simulink model "VTOL_renewal"  (R2023b)
settings: configuration reference "VTOLConfiguration" (kept outside this file)
undefined symbols (not defined in the file): CityMission, control, controlParams, ControlSampleTime, CriticalTiltAngle, DiscIntNeverNeededParam, env, F, FixedWingMission, flightState, FSState, FWControlParams, FWTrimSpeed, HoverMission, iniRoll, initPitch, iniYaw, Light, MIL, R_LOOKAHEAD, ReferenceFilterDen, ReferenceFilterNum, tilt_max, tilt_trim, tiltIni, TiltScheduleRate, TransitionMission, uavParam, vIni, Vt, w_trim, WindDownRate, windVel, xGround, yGround, zGround
libraries: slpidlib x56, simulink x6, uavalgslib x6, mbdriLib x4, aerolibasang x2, aerolibwind2 x2, shared6dof x1, sharedtransform x1, simulink_extras x1, sim3dlib x1, uavsim3dlib x1, uavutilslib x1
(part 2 of 8)

== system VTOL_renewal/Digital Twin/Ground Truth Bus ==
  Ve : Inport
  Xe : Inport  Port=2
  Euler : Inport  Port=3
  DCMbe : Inport  Port=4
  Vb : Inport  Port=5
  pqr : Inport  Port=6
  Abb : Inport  Port=7
  Abe : Inport  Port=8
  RotorParams : Inport  Port=9
  AirData : Inport  Port=10
  Bus Creator : BusCreator  Inputs=13
  Bus Selector : BusSelector  OutputSignals=airspeed
  Direction Cosine Matrix to Quaternions : sharedtransform/Direction Cosine Matrix  to Quaternions  aMode=0  action=None  tolerance=eps(2)
      settings: LibrarySourceBlock=|
      | aerolibtransform2/Direction Cosine Matrix
      | to Quaternions
  MATLAB Function1 : MATLAB Function  TreatAsAtomicUnit=on
  Ground Truth : Outport
  wires:
  pqr/1 -> Bus Creator/6
  Xe/1 -> Bus Creator/2
  Bus Creator/1 -> Ground Truth/1
  DCMbe/1 -> Direction Cosine Matrix to Quaternions/1, Bus Creator/4
  Euler/1 -> Bus Creator/3
  Vb/1 -> Bus Creator/5
  Abb/1 -> Bus Creator/7
  AirData/1 -> Bus Selector/1
  Bus Selector/1 -> Bus Creator/9  "<airspeed>"
  Direction Cosine Matrix to Quaternions/1 -> Bus Creator/10  "q"
  RotorParams/1 -> Bus Creator/8  "RotorParameters"
  Abe/1 -> Bus Creator/11  "Abe"
  MATLAB Function1/2(gndSpeed) -> Bus Creator/13  "gndspeed"
  MATLAB Function1/1(course) -> Bus Creator/12  "course"
  Ve/1 -> MATLAB Function1/1(vxyz), Bus Creator/1

== system VTOL_renewal/Digital Twin/Subsystem2 ==
  Euler : Inport
  pqr : Inport  Port=2
  Demux : Demux  Outputs=3
  Display : Display
  MATLAB Function : MATLAB Function  TreatAsAtomicUnit=on
  Matrix Multiply : Product  Multiplication=Matrix(*)
  Terminator : Terminator
  Euler Rate : Outport
  wires:
  Demux/1 -> MATLAB Function/1(phi)
  Demux/2 -> MATLAB Function/2(theta)
  MATLAB Function/1(y) -> Matrix Multiply/1
  pqr/1 -> Matrix Multiply/2
  Euler/1 -> Demux/1
  Demux/3 -> Terminator/1
  Matrix Multiply/1 -> Display/1, Euler Rate/1

== system VTOL_renewal/Guidance Test Bench/ControlType ==
  Aircraft States : Inport
  Global Mission : Inport  Port=2
  Guidance Testbench : Subsystem  TreatAsAtomicUnit=on  VariantControl=TestMode==1
  Manual Control : Subsystem  TreatAsAtomicUnit=on  VariantControl=TestMode==0
  HoverCmds : Outport
  FixedWingSP : Outport  Port=2
  AACSP : Outport  Port=3
  ctrlMode : Outport  Port=4
  FlightMode : Outport  Port=5

== system VTOL_renewal/Guidance Test Bench/Reference Tracking  ==
  State : Inport
  Position Command : Inport  Port=2
  AAC Commands : Inport  Port=3
  Fixed Wing Reference : Subsystem
  Hover Reference : Subsystem
  Transition Reference : Subsystem
  wires:
  State/1 -> Transition Reference/1(States), Fixed Wing Reference/2(States), Hover Reference/2(Position Reference)
  AAC Commands/1 -> Fixed Wing Reference/1(AAC Commands)
  Position Command/1 -> Hover Reference/1(Position Command)

== system VTOL_renewal/Visualization/No Visualization ==
  UAVState : Inport
  Terminator : Terminator
  wires:
  UAVState/1 -> Terminator/1

== system VTOL_renewal/Visualization/Photorealistic ==
  UAVState : Inport
  Bus Creator : BusCreator  Inputs=6
  Bus Selector : BusSelector  OutputSignals=Euler,Xe
  Demux : Demux  Outputs=3
  Demux1 : Demux  Outputs=3
  Prepare UAV Data : Subsystem
  Simulation 3D Scene Configuration : sim3dlib/Simulation 3D Scene Configuration  Priority=0  ProjectFormat=Unreal Editor  SceneDesc=US city block  ProjectName=I:\29\vdubey.MergedFixedWingReview\matlab\toolbox\shared\sim3d_projects\automotive_project_windows\UE\WindowsNoEditor\VehicleSimulation.exe  ScenePath=/Game/Maps/USCityBlock  UEProjPath=C:\Documents\project\AutoVrtlEnv\AutoVrtlEnv.uproject  EnableOpenDRIVE=off  vehTagList={'Scene Origin';'VTOL_Vehicle'}  vehTag=VTOL_Vehicle  FreeCameraInitialTranslation=[0, 0, 0]  FreeCameraDefaultInitialTranslation=[-6, 0, 2]  FreeCameraInitialRotation=[0, 0, 0]  FreeCameraDefaultInitialRotation=[0, -15, 0]  OpVisEn=off  Ts=1/10  EnableWindow=on  EnableRemoteAccess=off  EnableWeather=off  SunAltitude=40.0  SunAzimuth=90  clouds=10  wind=1  fog=0  rain=0  EnableGeospatial=off  OriginHeight=200  OriginLatitude=40.744652  OriginLongitude=-73.988864  MapStyle=Aerial  AdditionalAssetIDs=[]  UseAdvancedSunSky=off  SolarTime=11  TimeZone=-5  Day=21  Month=9  Year=2022  UseDaylightSavingTime=on  DSTStartDay=10  DSTStartMonth=3  DSTEndDay=3  DSTEndMonth=11  DSTSwitchHour=2  sensorTag=MainCamera2  sensorId=2  sensorName=MainCamera2  mountLoc=Origin  offsetFlag=off  tmountOffset=[0, 0, 0]  rmountOffset=[0, 0, 0]  HorizontalResolution=1280  VerticalResolution=720  HorizontalFOV=60  mountPoint=[0 0 0]  mountOrientation=[0 0 0]  aMode=4  ID=2  GeoTrigger=Inactive
      settings: LibrarySourceBlock=uavsim3dlib/Simulation 3D Scene Configuration
  Simulation 3D UAV Vehicle : uavsim3dlib/Simulation 3D UAV Vehicle  Priority=-1  Mesh=Custom  MeshPath=SkeletalMesh'/Game/Maps/VTOLDEMO/VTOLAsset.VTOLAsset'  Color=Black  ActorName=VTOL_Vehicle  UseGlobalFrame=off  InitialTranslation=[0 0 0]  InitialRotation=[0 0 0]  InitialTranslationGlobal=[0 0 0]  InitialGeoOrigin=[0 0 0]  InitialRotationGlobal=[0 0 0]  SampleTime=0.1  ActorType=SimulinkVehicle  ID=C  aMode=4  ActorTag=VTOL_Vehicle
  wires:
  UAVState/1 -> Bus Selector/1
  Bus Selector/2 -> Demux1/1  "<Xe>"
  Bus Selector/1 -> Demux/1  "<Euler>"
  Prepare UAV Data/2(Rotation) -> Simulation 3D UAV Vehicle/2
  Demux/1 -> Bus Creator/1  "roll"
  Demux/3 -> Bus Creator/3  "yaw"
  Demux1/1 -> Bus Creator/4  "x"
  Demux1/2 -> Bus Creator/5  "y"
  Bus Creator/1 -> Prepare UAV Data/1(UAVState)
  Demux1/3 -> Bus Creator/6  "z"
  Demux/2 -> Bus Creator/2  "pitch"
  Prepare UAV Data/1(Translation) -> Simulation 3D UAV Vehicle/1

== system VTOL_renewal/Visualization/Visualization ==
  UAVState : Inport
  Bus Selector : BusSelector  OutputSignals=Xe,q,RotorParameters.Rotor A,RotorParameters.Rotor B
  Gain : Gain  Gain=0
  Subsystem : Subsystem
  Trajectory : uavutilslib/UAV Animation  UAVType=FixedWing  UAVSize=5  InertialZDirection=Down  SampleTime=0.1
  wires:
  Bus Selector/2 -> Subsystem/2(<q>), Trajectory/2  "<q>"
  Bus Selector/1 -> Trajectory/1, Gain/1  "<Xe>"
  Gain/1 -> Subsystem/1(<Xe>)
  UAVState/1 -> Bus Selector/1
  Bus Selector/3 -> Subsystem/3(RotorA)  "<Rotor A>"
  Bus Selector/4 -> Subsystem/4(RotorB)  "<Rotor B>"

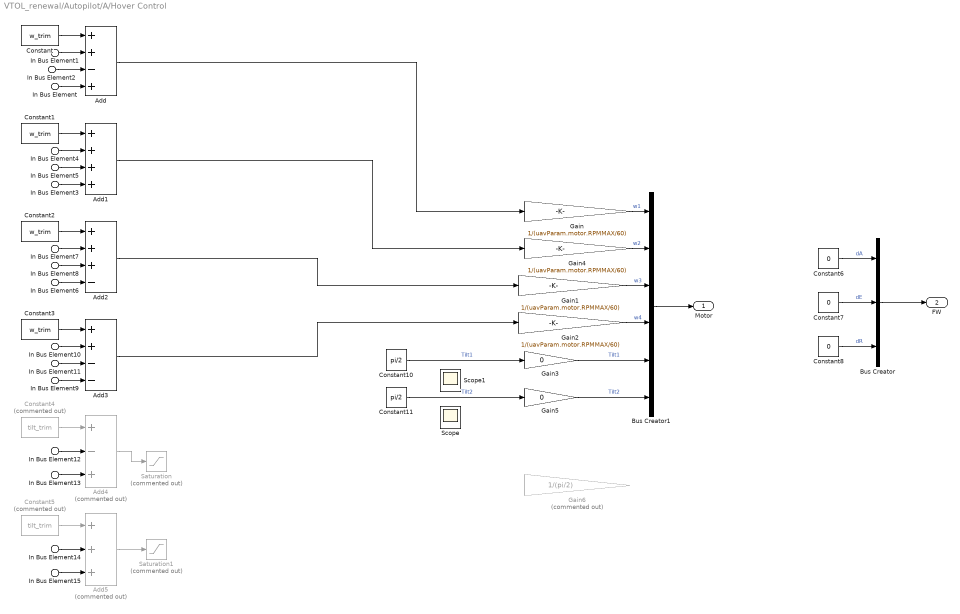
== system VTOL_renewal/Autopilot/A/Hover Control ==
  In Bus Element{,3,6,9} (4 alike) : Inport  PortName=MixerCommands  Element=w_theta
  In Bus Element{1,4,7,10} (4 alike) : Inport  PortName=MixerCommands  Element=w_z
  In Bus Element{2,5,8,11} (4 alike) : Inport  PortName=MixerCommands  Element=w_phi
  In Bus Element12 : Inport  PortName=MixerCommands  Element=l_psi
  In Bus Element14 : Inport  PortName=MixerCommands  Element=l_psi
  In Bus Element13 : Inport  PortName=MixerCommands  Element=l_x
  In Bus Element15 : Inport  PortName=MixerCommands  Element=l_x
  Add : Sum  Inputs=++-+
  Add1 : Sum  Inputs=++++
  Add2 : Sum  Inputs=+++-
  Add3 : Sum  Inputs=++--
  Add4 : Sum  Commented=on  Inputs=+-+
  Add5 : Sum  Commented=on  Inputs=+++
  Bus Creator : BusCreator  Inputs=3
  Bus Creator1 : BusCreator  Inputs=6  OutDataTypeStr=Bus: RotorCntrlBus
  Constant{,1..3} (4 alike) : Constant  Value=w_trim
  Constant10 : Constant  Value=pi/2
  Constant11 : Constant  Value=pi/2
  Constant4 : Constant  Commented=on  Value=tilt_trim
  Constant5 : Constant  Commented=on  Value=tilt_trim
  Constant6 : Constant  Value=0
  Constant7 : Constant  Value=0
  Constant8 : Constant  Value=0
  Gain{,1..2,4} (4 alike) : Gain  Gain=1/(uavParam.motor.RPMMAX/60)
  Gain3 : Gain  Gain=0
  Gain5 : Gain  Gain=0
  Gain6 : Gain  Commented=on  Gain=1/(pi/2)
  Saturation : Saturate  Commented=on  UpperLimit=tilt_max  LowerLimit=-tilt_max
  Saturation1 : Saturate  Commented=on  UpperLimit=tilt_max  LowerLimit=-tilt_max
  Scope : Scope
  Scope1 : Scope
  Motor : Outport
  FW : Outport  Port=2
  wires:
  In Bus Element4/1 -> Add1/2
  In Bus Element2/1 -> Add/3
  In Bus Element5/1 -> Add1/3
  Constant5/1 -> Add5/1
  In Bus Element3/1 -> Add1/4
  Add5/1 -> Saturation1/1
  In Bus Element/1 -> Add/4
  In Bus Element11/1 -> Add3/3
  In Bus Element8/1 -> Add2/3
  Constant2/1 -> Add2/1
  In Bus Element9/1 -> Add3/4
  In Bus Element6/1 -> Add2/4
  Constant1/1 -> Add1/1
  In Bus Element10/1 -> Add3/2
  In Bus Element1/1 -> Add/2
  Constant4/1 -> Add4/1
  Constant/1 -> Add/1
  Constant3/1 -> Add3/1
  Add4/1 -> Saturation/1
  In Bus Element7/1 -> Add2/2
  In Bus Element12/1 -> Add4/2
  In Bus Element13/1 -> Add4/3
  In Bus Element14/1 -> Add5/2
  In Bus Element15/1 -> Add5/3
  Bus Creator/1 -> FW/1
  Constant6/1 -> Bus Creator/1  "dA"
  Constant7/1 -> Bus Creator/2  "dE"
  Constant8/1 -> Bus Creator/3  "dR"
  Bus Creator1/1 -> Motor/1
  Constant11/1 -> Gain5/1  "Tilt2"
  Gain2/1 -> Bus Creator1/4  "w4"
  Add/1 -> Gain/1
  Gain/1 -> Bus Creator1/1  "w1"
  Constant10/1 -> Gain3/1  "Tilt1"
  Gain1/1 -> Bus Creator1/3  "w3"
  Add3/1 -> Gain2/1
  Add1/1 -> Gain4/1
  Gain4/1 -> Bus Creator1/2  "w2"
  Add2/1 -> Gain1/1
  Gain3/1 -> Bus Creator1/5  "Tilt1"
  Gain5/1 -> Bus Creator1/6  "Tilt2"

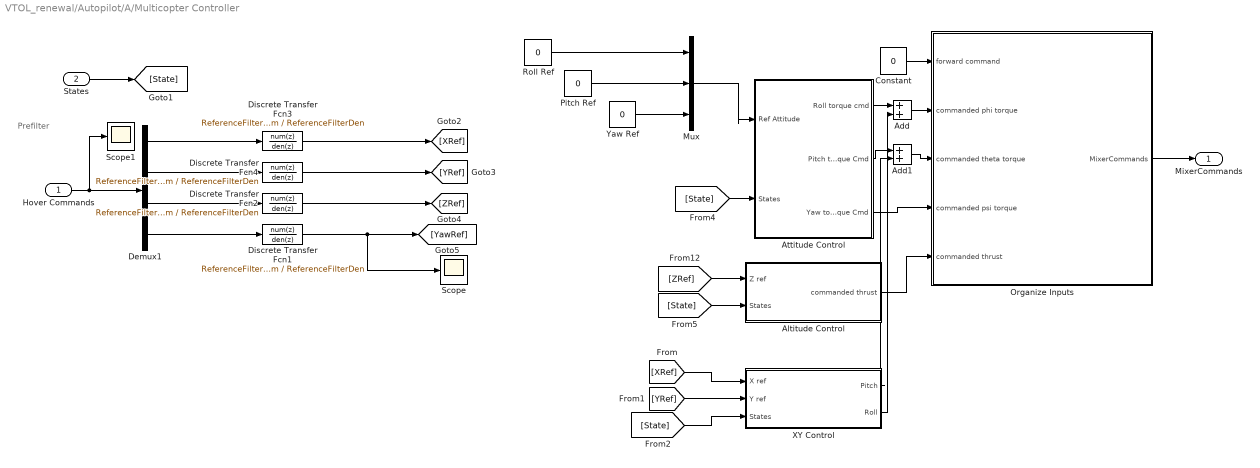
== system VTOL_renewal/Autopilot/A/Multicopter Controller ==
  note: Prefilter
  Hover Commands : Inport
  States : Inport  Port=2
  Add : Sum
  Add1 : Sum
  Altitude Control : Subsystem
  Attitude Control : Subsystem
  Constant : Constant  Value=0
  Demux1 : Demux
  Discrete Transfer Fcn{1..4} (4 alike) : DiscreteTransferFcn  Numerator=ReferenceFilterNum  Denominator=ReferenceFilterDen
  Mux : Mux  Inputs=3
  Organize Inputs : Subsystem
  Pitch Ref : Constant  Value=0
  Roll Ref : Constant  Value=0
  Scope : Scope
  Scope1 : Scope
  XY Control : Subsystem
  Yaw Ref : Constant  Value=0
  MixerCommands : Outport
  wires:
  Roll Ref/1 -> Mux/1
  States/1 -> [State]
  Hover Commands/1 -> Demux1/1, Scope1/1
  Attitude Control/1(Roll torque cmd) -> Add/1
  Demux1/3 -> Discrete Transfer Fcn2/1
  Demux1/1 -> Discrete Transfer Fcn3/1
  [State] -> Altitude Control/2(States)
  Demux1/2 -> Discrete Transfer Fcn4/1
  Discrete Transfer Fcn3/1 -> [XRef]
  Demux1/4 -> Discrete Transfer Fcn1/1
  Attitude Control/3(Yaw torque Cmd) -> Organize Inputs/4(commanded psi torque)
  Discrete Transfer Fcn4/1 -> [YRef]
  Constant/1 -> Organize Inputs/1(forward command)
  Pitch Ref/1 -> Mux/2
  Yaw Ref/1 -> Mux/3
  Mux/1 -> Attitude Control/1(Ref Attitude)
  [State] -> Attitude Control/2(States)
  [ZRef] -> Altitude Control/1(Z ref)
  Altitude Control/1(commanded thrust) -> Organize Inputs/5(commanded thrust)
  Organize Inputs/1(MixerCommands) -> MixerCommands/1
  Discrete Transfer Fcn1/1 -> Scope/1, [YawRef]
  Discrete Transfer Fcn2/1 -> [ZRef]
  [XRef] -> XY Control/1(X ref)
  [YRef] -> XY Control/2(Y ref)
  [State] -> XY Control/3(States)
  Add/1 -> Organize Inputs/2(commanded phi torque)
  XY Control/2(Roll) -> Add/2
  XY Control/1(Pitch) -> Add1/2
  Attitude Control/2(Pitch torque Cmd) -> Add1/1
  Add1/1 -> Organize Inputs/3(commanded theta torque)

== system VTOL_renewal/Autopilot/B/Subsystem2 ==
  Euler : Inport
  pqr : Inport  Port=2
  Demux : Demux  Outputs=3
  Display : Display
  MATLAB Function : MATLAB Function  TreatAsAtomicUnit=on
  Matrix Multiply : Product  Multiplication=Matrix(*)
  Terminator : Terminator
  Euler Rate : Outport
  wires:
  Demux/1 -> MATLAB Function/1(phi)
  Demux/2 -> MATLAB Function/2(theta)
  MATLAB Function/1(y) -> Matrix Multiply/1
  pqr/1 -> Matrix Multiply/2
  Euler/1 -> Demux/1
  Demux/3 -> Terminator/1
  Matrix Multiply/1 -> Display/1, Euler Rate/1

== system VTOL_renewal/Autopilot/C/Actuator To Voltage1 ==
  Motor Commands : Inport
  Bus Creator : BusCreator  Inputs=6  OutDataTypeStr=Bus: RotorCntrlBus
  Bus Selector : BusSelector  OutputSignals=w1,w2,w3,w4,Tilt1,Tilt2
  Gain{,1..2,4} (4 alike) : Gain  Gain=1/(uavParam.motor.RPMMAX/60)
  Gain3 : Gain  Gain=1/(pi/2)
  Gain5 : Gain  Gain=1/(pi/2)
  To PWM : Outport
  wires:
  Motor Commands/1 -> Bus Selector/1
  Bus Selector/1 -> Gain/1  "<w1>"
  Bus Selector/3 -> Gain1/1  "<w3>"
  Bus Selector/2 -> Gain4/1  "<w2>"
  Bus Selector/4 -> Gain2/1  "<w4>"
  Bus Selector/5 -> Gain3/1  "<Tilt1>"
  Bus Selector/6 -> Gain5/1  "<Tilt2>"
  Gain/1 -> Bus Creator/1  "w1"
  Gain4/1 -> Bus Creator/2  "w2"
  Gain1/1 -> Bus Creator/3  "w3"
  Gain2/1 -> Bus Creator/4  "w4"
  Gain3/1 -> Bus Creator/5  "Tilt1"
  Gain5/1 -> Bus Creator/6  "Tilt2"
  Bus Creator/1 -> To PWM/1

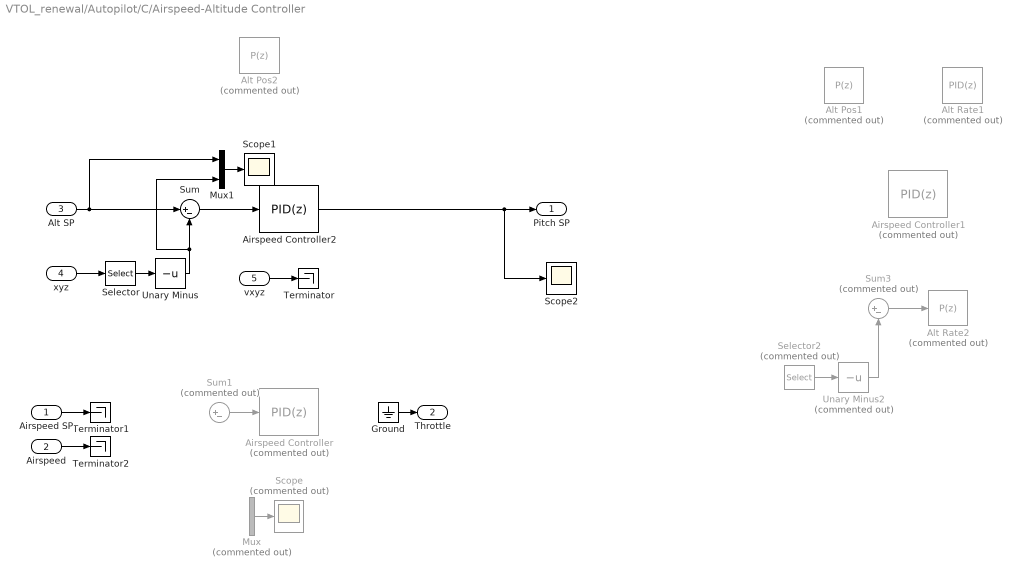
== system VTOL_renewal/Autopilot/C/Airspeed-Altitude Controller ==
  Airspeed SP : Inport
  Airspeed : Inport  Port=2
  Alt SP : Inport  Port=3
  xyz : Inport  Port=4
  vxyz : Inport  Port=5
  Airspeed Controller : slpidlib/PID Controller  Commented=on  Controller=PID  Form=Parallel  TimeDomain=Discrete-time  UseExternalTs=off  SampleTime=ControlSampleTime  IntegratorMethod=Trapezoidal  FilterMethod=Forward Euler  ControllerParametersSource=internal  P=FWControlParams.P_AIRSPD  I=FWControlParams.I_AIRSPD  UseKiTs=off  D=FWControlParams.D_AIRSPD  N=FWControlParams.N_AIRSPD  UseFilter=on  TunerSelectOption=Transfer Function Based (PID Tuner App)  InitialConditionSource=internal  InitialConditionForIntegrator=0  InitialConditionForFilter=0  DifferentiatorICPrevScaledInput=0  ExternalReset=none  TrackingMode=off  Kt=1  LimitOutput=off  SatLimitsSource=internal  UpperSaturationLimit=Inf  LowerSaturationLimit=0  LinearizeAsGain=on  AntiWindupMode=clamping  Kb=1  LimitIntegrator=off  UpperIntegratorSaturationLimit=inf  LowerIntegratorSaturationLimit=-inf  POutMin=[]  POutMax=[]  IOutMin=[]  IOutMax=[]  DOutMin=[]  DOutMax=[]  NOutMin=[]  NOutMax=[]  SumOutMin=[]  SumOutMax=[]  SaturationOutMin=[]  SaturationOutMax=[]  PParamMin=[]  PParamMax=[]  IParamMin=[]  IParamMax=[]  DParamMin=[]  DParamMax=[]  NParamMin=[]  NParamMax=[]  KbParamMin=[]  KbParamMax=[]  KtParamMin=[]  KtParamMax=[]  KbOutMin=[]  KbOutMax=[]  KtOutMin=[]  KtOutMax=[]  IntegratorOutMin=[]  IntegratorOutMax=[]  FilterOutMin=[]  FilterOutMax=[]  SumI1OutMin=[]  SumI1OutMax=[]  SumI2OutMin=[]  SumI2OutMax=[]  SumI3OutMin=[]  SumI3OutMax=[]  SumI4OutMin=[]  SumI4OutMax=[]  SumDOutMin=[]  SumDOutMax=[]  DifferentiatorOutMin=[]  DifferentiatorOutMax=[]  FilterDiffOutCoefMin=[]  FilterDiffOutCoefMax=[]  ReciprocalOutMin=[]  ReciprocalOutMax=[]  SumDenOutMin=[]  SumDenOutMax=[]  SumNumOutMin=[]  SumNumOutMax=[]  DivideOutMin=[]  DivideOutMax=[]  UdiffTsProdOutMin=[]  UdiffTsProdOutMax=[]  NTsProdOutMin=[]  NTsProdOutMax=[]  UintegralTsProdOutMin=[]  UintegralTsProdOutMax=[]  UngainTsProdOutMin=[]  UngainTsProdOutMax=[]  ClampingZeroOutDataTypeStr=Inherit: Inherit via back propagation  ClampingZeroOutMin=[]  ClampingZeroOutMax=[]  FilterDenConstantOutDataTypeStr=Inherit: Inherit via back propagation  FilterDenConstantOutMin=[]  FilterDenConstantOutMax=[]  PCopyOutDataTypeStr=Inherit: Inherit via back propagation  PCopyOutMin=[]  PCopyOutMax=[]  NCopyOutDataTypeStr=Inherit: Inherit via back propagation  NCopyOutMin=[]  NCopyOutMax=[]  IntegratorContinuousStateAttributes=''  IntegratorStateMustResolveToSignalObject=off  IntegratorRTWStateStorageClass=Auto  FilterContinuousStateAttributes=''  FilterStateMustResolveToSignalObject=off  FilterRTWStateStorageClass=Auto  ParallelPVariant=InternalParameters  IdealPVariant=Disabled  IVariant=InternalParameters  DVariant=InternalParameters  IntegratorVariant=Discrete  SatVariant=Disabled  AWVariant=Passthrough  PCopyVariant=Disabled  TRVariant=Disabled  FdbkBlocksVariant=Forward  IdealPFdbkVariant=Disabled  SatFdbkVariant=Disabled  DerivativeFilterVariant=ForwardEulerFilter  NVariant=InternalParameters  NCopyVariant=Disabled  FilterICVariant=InternalICsFilter  IntegratorICVariant=InternalICs  ExternalResetVariant=Disabled  TRSumVariant=Passthrough  SumFdbkVariant=Disabled  SumVariant=Sum_PID  TsampFilterVariant=InternalTs  TsampNgainVariant=Passthrough  TsampIntegralVariant=Disabled_SignalSpec  ExternalSaturationOutDataTypeStr=Inherit: Same as second input
  Airspeed Controller1 : slpidlib/PID Controller  Commented=on  Controller=PID  Form=Parallel  TimeDomain=Discrete-time  UseExternalTs=off  SampleTime=ControlSampleTime  IntegratorMethod=Trapezoidal  FilterMethod=Forward Euler  ControllerParametersSource=internal  P=FWControlParams.P_AIRSPD  I=FWControlParams.I_AIRSPD  UseKiTs=off  D=FWControlParams.D_AIRSPD  N=FWControlParams.N_AIRSPD  UseFilter=on  TunerSelectOption=Transfer Function Based (PID Tuner App)  InitialConditionSource=internal  InitialConditionForIntegrator=0  InitialConditionForFilter=0  DifferentiatorICPrevScaledInput=0  ExternalReset=none  TrackingMode=off  Kt=1  LimitOutput=off  SatLimitsSource=internal  UpperSaturationLimit=Inf  LowerSaturationLimit=0  LinearizeAsGain=on  AntiWindupMode=clamping  Kb=1  LimitIntegrator=off  UpperIntegratorSaturationLimit=inf  LowerIntegratorSaturationLimit=-inf  POutMin=[]  POutMax=[]  IOutMin=[]  IOutMax=[]  DOutMin=[]  DOutMax=[]  NOutMin=[]  NOutMax=[]  SumOutMin=[]  SumOutMax=[]  SaturationOutMin=[]  SaturationOutMax=[]  PParamMin=[]  PParamMax=[]  IParamMin=[]  IParamMax=[]  DParamMin=[]  DParamMax=[]  NParamMin=[]  NParamMax=[]  KbParamMin=[]  KbParamMax=[]  KtParamMin=[]  KtParamMax=[]  KbOutMin=[]  KbOutMax=[]  KtOutMin=[]  KtOutMax=[]  IntegratorOutMin=[]  IntegratorOutMax=[]  FilterOutMin=[]  FilterOutMax=[]  SumI1OutMin=[]  SumI1OutMax=[]  SumI2OutMin=[]  SumI2OutMax=[]  SumI3OutMin=[]  SumI3OutMax=[]  SumI4OutMin=[]  SumI4OutMax=[]  SumDOutMin=[]  SumDOutMax=[]  DifferentiatorOutMin=[]  DifferentiatorOutMax=[]  FilterDiffOutCoefMin=[]  FilterDiffOutCoefMax=[]  ReciprocalOutMin=[]  ReciprocalOutMax=[]  SumDenOutMin=[]  SumDenOutMax=[]  SumNumOutMin=[]  SumNumOutMax=[]  DivideOutMin=[]  DivideOutMax=[]  UdiffTsProdOutMin=[]  UdiffTsProdOutMax=[]  NTsProdOutMin=[]  NTsProdOutMax=[]  UintegralTsProdOutMin=[]  UintegralTsProdOutMax=[]  UngainTsProdOutMin=[]  UngainTsProdOutMax=[]  ClampingZeroOutDataTypeStr=Inherit: Inherit via back propagation  ClampingZeroOutMin=[]  ClampingZeroOutMax=[]  FilterDenConstantOutDataTypeStr=Inherit: Inherit via back propagation  FilterDenConstantOutMin=[]  FilterDenConstantOutMax=[]  PCopyOutDataTypeStr=Inherit: Inherit via back propagation  PCopyOutMin=[]  PCopyOutMax=[]  NCopyOutDataTypeStr=Inherit: Inherit via back propagation  NCopyOutMin=[]  NCopyOutMax=[]  IntegratorContinuousStateAttributes=''  IntegratorStateMustResolveToSignalObject=off  IntegratorRTWStateStorageClass=Auto  FilterContinuousStateAttributes=''  FilterStateMustResolveToSignalObject=off  FilterRTWStateStorageClass=Auto  ParallelPVariant=InternalParameters  IdealPVariant=Disabled  IVariant=InternalParameters  DVariant=InternalParameters  IntegratorVariant=Discrete  SatVariant=Disabled  AWVariant=Passthrough  PCopyVariant=Disabled  TRVariant=Disabled  FdbkBlocksVariant=Forward  IdealPFdbkVariant=Disabled  SatFdbkVariant=Disabled  DerivativeFilterVariant=ForwardEulerFilter  NVariant=InternalParameters  NCopyVariant=Disabled  FilterICVariant=InternalICsFilter  IntegratorICVariant=InternalICs  ExternalResetVariant=Disabled  TRSumVariant=Passthrough  SumFdbkVariant=Disabled  SumVariant=Sum_PID  TsampFilterVariant=InternalTs  TsampNgainVariant=Passthrough  TsampIntegralVariant=Disabled_SignalSpec  ExternalSaturationOutDataTypeStr=Inherit: Same as second input
  Airspeed Controller2 : slpidlib/PID Controller  Controller=PID  Form=Parallel  TimeDomain=Discrete-time  UseExternalTs=off  SampleTime=ControlSampleTime  IntegratorMethod=Trapezoidal  FilterMethod=Forward Euler  ControllerParametersSource=internal  P=10  I=1  UseKiTs=off  D=0  N=FWControlParams.N_AIRSPD  UseFilter=on  TunerSelectOption=Transfer Function Based (PID Tuner App)  InitialConditionSource=internal  InitialConditionForIntegrator=0  InitialConditionForFilter=0  DifferentiatorICPrevScaledInput=0  ExternalReset=none  TrackingMode=off  Kt=1  LimitOutput=off  SatLimitsSource=internal  UpperSaturationLimit=Inf  LowerSaturationLimit=0  LinearizeAsGain=on  AntiWindupMode=clamping  Kb=1  LimitIntegrator=off  UpperIntegratorSaturationLimit=inf  LowerIntegratorSaturationLimit=-inf  POutMin=[]  POutMax=[]  IOutMin=[]  IOutMax=[]  DOutMin=[]  DOutMax=[]  NOutMin=[]  NOutMax=[]  SumOutMin=[]  SumOutMax=[]  SaturationOutMin=[]  SaturationOutMax=[]  PParamMin=[]  PParamMax=[]  IParamMin=[]  IParamMax=[]  DParamMin=[]  DParamMax=[]  NParamMin=[]  NParamMax=[]  KbParamMin=[]  KbParamMax=[]  KtParamMin=[]  KtParamMax=[]  KbOutMin=[]  KbOutMax=[]  KtOutMin=[]  KtOutMax=[]  IntegratorOutMin=[]  IntegratorOutMax=[]  FilterOutMin=[]  FilterOutMax=[]  SumI1OutMin=[]  SumI1OutMax=[]  SumI2OutMin=[]  SumI2OutMax=[]  SumI3OutMin=[]  SumI3OutMax=[]  SumI4OutMin=[]  SumI4OutMax=[]  SumDOutMin=[]  SumDOutMax=[]  DifferentiatorOutMin=[]  DifferentiatorOutMax=[]  FilterDiffOutCoefMin=[]  FilterDiffOutCoefMax=[]  ReciprocalOutMin=[]  ReciprocalOutMax=[]  SumDenOutMin=[]  SumDenOutMax=[]  SumNumOutMin=[]  SumNumOutMax=[]  DivideOutMin=[]  DivideOutMax=[]  UdiffTsProdOutMin=[]  UdiffTsProdOutMax=[]  NTsProdOutMin=[]  NTsProdOutMax=[]  UintegralTsProdOutMin=[]  UintegralTsProdOutMax=[]  UngainTsProdOutMin=[]  UngainTsProdOutMax=[]  ClampingZeroOutDataTypeStr=Inherit: Inherit via back propagation  ClampingZeroOutMin=[]  ClampingZeroOutMax=[]  FilterDenConstantOutDataTypeStr=Inherit: Inherit via back propagation  FilterDenConstantOutMin=[]  FilterDenConstantOutMax=[]  PCopyOutDataTypeStr=Inherit: Inherit via back propagation  PCopyOutMin=[]  PCopyOutMax=[]  NCopyOutDataTypeStr=Inherit: Inherit via back propagation  NCopyOutMin=[]  NCopyOutMax=[]  IntegratorContinuousStateAttributes=''  IntegratorStateMustResolveToSignalObject=off  IntegratorRTWStateStorageClass=Auto  FilterContinuousStateAttributes=''  FilterStateMustResolveToSignalObject=off  FilterRTWStateStorageClass=Auto  ParallelPVariant=InternalParameters  IdealPVariant=Disabled  IVariant=InternalParameters  DVariant=InternalParameters  IntegratorVariant=Discrete  SatVariant=Disabled  AWVariant=Passthrough  PCopyVariant=Disabled  TRVariant=Disabled  FdbkBlocksVariant=Forward  IdealPFdbkVariant=Disabled  SatFdbkVariant=Disabled  DerivativeFilterVariant=ForwardEulerFilter  NVariant=InternalParameters  NCopyVariant=Disabled  FilterICVariant=InternalICsFilter  IntegratorICVariant=InternalICs  ExternalResetVariant=Disabled  TRSumVariant=Passthrough  SumFdbkVariant=Disabled  SumVariant=Sum_PID  TsampFilterVariant=InternalTs  TsampNgainVariant=Passthrough  TsampIntegralVariant=Disabled_SignalSpec  ExternalSaturationOutDataTypeStr=Inherit: Same as second input
  Alt Pos1 : slpidlib/PID Controller  Commented=on  Controller=P  Form=Parallel  TimeDomain=Discrete-time  UseExternalTs=off  SampleTime=-1  IntegratorMethod=Forward Euler  FilterMethod=Forward Euler  ControllerParametersSource=internal  P=FWControlParams.P_ALT  I=0  UseKiTs=off  D=0  N=100  UseFilter=on  TunerSelectOption=Transfer Function Based (PID Tuner App)  InitialConditionSource=internal  InitialConditionForIntegrator=0  InitialConditionForFilter=0  DifferentiatorICPrevScaledInput=0  ExternalReset=none  TrackingMode=off  Kt=1  LimitOutput=on  SatLimitsSource=internal  UpperSaturationLimit=control.maxClimbRate  LowerSaturationLimit=control.maxDescendRate  LinearizeAsGain=on  AntiWindupMode=clamping  Kb=1  LimitIntegrator=off  UpperIntegratorSaturationLimit=inf  LowerIntegratorSaturationLimit=-inf  POutMin=[]  POutMax=[]  IOutMin=[]  IOutMax=[]  DOutMin=[]  DOutMax=[]  NOutMin=[]  NOutMax=[]  SumOutMin=[]  SumOutMax=[]  SaturationOutMin=[]  SaturationOutMax=[]  PParamMin=[]  PParamMax=[]  IParamMin=[]  IParamMax=[]  DParamMin=[]  DParamMax=[]  NParamMin=[]  NParamMax=[]  KbParamMin=[]  KbParamMax=[]  KtParamMin=[]  KtParamMax=[]  KbOutMin=[]  KbOutMax=[]  KtOutMin=[]  KtOutMax=[]  IntegratorOutMin=[]  IntegratorOutMax=[]  FilterOutMin=[]  FilterOutMax=[]  SumI1OutMin=[]  SumI1OutMax=[]  SumI2OutMin=[]  SumI2OutMax=[]  SumI3OutMin=[]  SumI3OutMax=[]  SumI4OutMin=[]  SumI4OutMax=[]  SumDOutMin=[]  SumDOutMax=[]  DifferentiatorOutMin=[]  DifferentiatorOutMax=[]  FilterDiffOutCoefMin=[]  FilterDiffOutCoefMax=[]  ReciprocalOutMin=[]  ReciprocalOutMax=[]  SumDenOutMin=[]  SumDenOutMax=[]  SumNumOutMin=[]  SumNumOutMax=[]  DivideOutMin=[]  DivideOutMax=[]  UdiffTsProdOutMin=[]  UdiffTsProdOutMax=[]  NTsProdOutMin=[]  NTsProdOutMax=[]  UintegralTsProdOutMin=[]  UintegralTsProdOutMax=[]  UngainTsProdOutMin=[]  UngainTsProdOutMax=[]  ClampingZeroOutDataTypeStr=Inherit: Inherit via back propagation  ClampingZeroOutMin=[]  ClampingZeroOutMax=[]  FilterDenConstantOutDataTypeStr=Inherit: Inherit via back propagation  FilterDenConstantOutMin=[]  FilterDenConstantOutMax=[]  PCopyOutDataTypeStr=Inherit: Inherit via back propagation  PCopyOutMin=[]  PCopyOutMax=[]  NCopyOutDataTypeStr=Inherit: Inherit via back propagation  NCopyOutMin=[]  NCopyOutMax=[]  IntegratorContinuousStateAttributes=''  IntegratorStateMustResolveToSignalObject=off  IntegratorRTWStateStorageClass=Auto  FilterContinuousStateAttributes=''  FilterStateMustResolveToSignalObject=off  FilterRTWStateStorageClass=Auto  ParallelPVariant=InternalParameters  IdealPVariant=Disabled  IVariant=Disabled  DVariant=Disabled  IntegratorVariant=Disabled  SatVariant=Enabled  AWVariant=Disabled  PCopyVariant=Disabled  TRVariant=Disabled  FdbkBlocksVariant=Forward  IdealPFdbkVariant=Disabled  SatFdbkVariant=Disabled  DerivativeFilterVariant=Disabled  NVariant=Disabled  NCopyVariant=Disabled_SignalSpec  FilterICVariant=Disabled  IntegratorICVariant=Disabled  ExternalResetVariant=Disabled  TRSumVariant=Passthrough  SumFdbkVariant=Disabled  SumVariant=Passthrough_P  TsampFilterVariant=InternalTs  TsampNgainVariant=Passthrough  TsampIntegralVariant=Disabled_SignalSpec  ExternalSaturationOutDataTypeStr=Inherit: Same as second input
  Alt Pos2 : slpidlib/PID Controller  Commented=on  Controller=P  Form=Parallel  TimeDomain=Discrete-time  UseExternalTs=off  SampleTime=-1  IntegratorMethod=Forward Euler  FilterMethod=Forward Euler  ControllerParametersSource=internal  P=FWControlParams.P_ALT  I=0  UseKiTs=off  D=0  N=100  UseFilter=on  TunerSelectOption=Transfer Function Based (PID Tuner App)  InitialConditionSource=internal  InitialConditionForIntegrator=0  InitialConditionForFilter=0  DifferentiatorICPrevScaledInput=0  ExternalReset=none  TrackingMode=off  Kt=1  LimitOutput=on  SatLimitsSource=internal  UpperSaturationLimit=control.maxClimbRate  LowerSaturationLimit=control.maxDescendRate  LinearizeAsGain=on  AntiWindupMode=clamping  Kb=1  LimitIntegrator=off  UpperIntegratorSaturationLimit=inf  LowerIntegratorSaturationLimit=-inf  POutMin=[]  POutMax=[]  IOutMin=[]  IOutMax=[]  DOutMin=[]  DOutMax=[]  NOutMin=[]  NOutMax=[]  SumOutMin=[]  SumOutMax=[]  SaturationOutMin=[]  SaturationOutMax=[]  PParamMin=[]  PParamMax=[]  IParamMin=[]  IParamMax=[]  DParamMin=[]  DParamMax=[]  NParamMin=[]  NParamMax=[]  KbParamMin=[]  KbParamMax=[]  KtParamMin=[]  KtParamMax=[]  KbOutMin=[]  KbOutMax=[]  KtOutMin=[]  KtOutMax=[]  IntegratorOutMin=[]  IntegratorOutMax=[]  FilterOutMin=[]  FilterOutMax=[]  SumI1OutMin=[]  SumI1OutMax=[]  SumI2OutMin=[]  SumI2OutMax=[]  SumI3OutMin=[]  SumI3OutMax=[]  SumI4OutMin=[]  SumI4OutMax=[]  SumDOutMin=[]  SumDOutMax=[]  DifferentiatorOutMin=[]  DifferentiatorOutMax=[]  FilterDiffOutCoefMin=[]  FilterDiffOutCoefMax=[]  ReciprocalOutMin=[]  ReciprocalOutMax=[]  SumDenOutMin=[]  SumDenOutMax=[]  SumNumOutMin=[]  SumNumOutMax=[]  DivideOutMin=[]  DivideOutMax=[]  UdiffTsProdOutMin=[]  UdiffTsProdOutMax=[]  NTsProdOutMin=[]  NTsProdOutMax=[]  UintegralTsProdOutMin=[]  UintegralTsProdOutMax=[]  UngainTsProdOutMin=[]  UngainTsProdOutMax=[]  ClampingZeroOutDataTypeStr=Inherit: Inherit via back propagation  ClampingZeroOutMin=[]  ClampingZeroOutMax=[]  FilterDenConstantOutDataTypeStr=Inherit: Inherit via back propagation  FilterDenConstantOutMin=[]  FilterDenConstantOutMax=[]  PCopyOutDataTypeStr=Inherit: Inherit via back propagation  PCopyOutMin=[]  PCopyOutMax=[]  NCopyOutDataTypeStr=Inherit: Inherit via back propagation  NCopyOutMin=[]  NCopyOutMax=[]  IntegratorContinuousStateAttributes=''  IntegratorStateMustResolveToSignalObject=off  IntegratorRTWStateStorageClass=Auto  FilterContinuousStateAttributes=''  FilterStateMustResolveToSignalObject=off  FilterRTWStateStorageClass=Auto  ParallelPVariant=InternalParameters  IdealPVariant=Disabled  IVariant=Disabled  DVariant=Disabled  IntegratorVariant=Disabled  SatVariant=Enabled  AWVariant=Disabled  PCopyVariant=Disabled  TRVariant=Disabled  FdbkBlocksVariant=Forward  IdealPFdbkVariant=Disabled  SatFdbkVariant=Disabled  DerivativeFilterVariant=Disabled  NVariant=Disabled  NCopyVariant=Disabled_SignalSpec  FilterICVariant=Disabled  IntegratorICVariant=Disabled  ExternalResetVariant=Disabled  TRSumVariant=Passthrough  SumFdbkVariant=Disabled  SumVariant=Passthrough_P  TsampFilterVariant=InternalTs  TsampNgainVariant=Passthrough  TsampIntegralVariant=Disabled_SignalSpec  ExternalSaturationOutDataTypeStr=Inherit: Same as second input
  Alt Rate1 : slpidlib/PID Controller  Commented=on  Controller=PID  Form=Parallel  TimeDomain=Discrete-time  UseExternalTs=off  SampleTime=-1  IntegratorMethod=Forward Euler  FilterMethod=Forward Euler  ControllerParametersSource=internal  P=FWControlParams.P_CLIMBRATE  I=0  UseKiTs=off  D=0  N=100  UseFilter=on  TunerSelectOption=Transfer Function Based (PID Tuner App)  InitialConditionSource=internal  InitialConditionForIntegrator=0  InitialConditionForFilter=0  DifferentiatorICPrevScaledInput=0  ExternalReset=none  TrackingMode=off  Kt=1  LimitOutput=on  SatLimitsSource=internal  UpperSaturationLimit=control.maxPitch  LowerSaturationLimit=control.minPitch  LinearizeAsGain=on  AntiWindupMode=clamping  Kb=1  LimitIntegrator=off  UpperIntegratorSaturationLimit=inf  LowerIntegratorSaturationLimit=-inf  POutMin=[]  POutMax=[]  IOutMin=[]  IOutMax=[]  DOutMin=[]  DOutMax=[]  NOutMin=[]  NOutMax=[]  SumOutMin=[]  SumOutMax=[]  SaturationOutMin=[]  SaturationOutMax=[]  PParamMin=[]  PParamMax=[]  IParamMin=[]  IParamMax=[]  DParamMin=[]  DParamMax=[]  NParamMin=[]  NParamMax=[]  KbParamMin=[]  KbParamMax=[]  KtParamMin=[]  KtParamMax=[]  KbOutMin=[]  KbOutMax=[]  KtOutMin=[]  KtOutMax=[]  IntegratorOutMin=[]  IntegratorOutMax=[]  FilterOutMin=[]  FilterOutMax=[]  SumI1OutMin=[]  SumI1OutMax=[]  SumI2OutMin=[]  SumI2OutMax=[]  SumI3OutMin=[]  SumI3OutMax=[]  SumI4OutMin=[]  SumI4OutMax=[]  SumDOutMin=[]  SumDOutMax=[]  DifferentiatorOutMin=[]  DifferentiatorOutMax=[]  FilterDiffOutCoefMin=[]  FilterDiffOutCoefMax=[]  ReciprocalOutMin=[]  ReciprocalOutMax=[]  SumDenOutMin=[]  SumDenOutMax=[]  SumNumOutMin=[]  SumNumOutMax=[]  DivideOutMin=[]  DivideOutMax=[]  UdiffTsProdOutMin=[]  UdiffTsProdOutMax=[]  NTsProdOutMin=[]  NTsProdOutMax=[]  UintegralTsProdOutMin=[]  UintegralTsProdOutMax=[]  UngainTsProdOutMin=[]  UngainTsProdOutMax=[]  ClampingZeroOutDataTypeStr=Inherit: Inherit via back propagation  ClampingZeroOutMin=[]  ClampingZeroOutMax=[]  FilterDenConstantOutDataTypeStr=Inherit: Inherit via back propagation  FilterDenConstantOutMin=[]  FilterDenConstantOutMax=[]  PCopyOutDataTypeStr=Inherit: Inherit via back propagation  PCopyOutMin=[]  PCopyOutMax=[]  NCopyOutDataTypeStr=Inherit: Inherit via back propagation  NCopyOutMin=[]  NCopyOutMax=[]  IntegratorContinuousStateAttributes=''  IntegratorStateMustResolveToSignalObject=off  IntegratorRTWStateStorageClass=Auto  FilterContinuousStateAttributes=''  FilterStateMustResolveToSignalObject=off  FilterRTWStateStorageClass=Auto  ParallelPVariant=InternalParameters  IdealPVariant=Disabled  IVariant=InternalParameters  DVariant=InternalParameters  IntegratorVariant=Discrete  SatVariant=Enabled  AWVariant=DiscClampingParallel  PCopyVariant=Disabled  TRVariant=Disabled  FdbkBlocksVariant=Forward  IdealPFdbkVariant=Disabled  SatFdbkVariant=Disabled  DerivativeFilterVariant=ForwardEulerFilter  NVariant=InternalParameters  NCopyVariant=Disabled  FilterICVariant=InternalICsFilter  IntegratorICVariant=InternalICs  ExternalResetVariant=Disabled  TRSumVariant=Passthrough  SumFdbkVariant=Disabled  SumVariant=Sum_PID  TsampFilterVariant=InternalTs  TsampNgainVariant=Passthrough  TsampIntegralVariant=Disabled_SignalSpec  ExternalSaturationOutDataTypeStr=Inherit: Same as second input
  Alt Rate2 : slpidlib/PID Controller  Commented=on  Controller=P  Form=Parallel  TimeDomain=Discrete-time  UseExternalTs=off  SampleTime=-1  IntegratorMethod=Forward Euler  FilterMethod=Forward Euler  ControllerParametersSource=internal  P=FWControlParams.P_CLIMBRATE  I=0  UseKiTs=off  D=0  N=100  UseFilter=on  TunerSelectOption=Transfer Function Based (PID Tuner App)  InitialConditionSource=internal  InitialConditionForIntegrator=0  InitialConditionForFilter=0  DifferentiatorICPrevScaledInput=0  ExternalReset=none  TrackingMode=off  Kt=1  LimitOutput=on  SatLimitsSource=internal  UpperSaturationLimit=control.maxPitch  LowerSaturationLimit=control.minPitch  LinearizeAsGain=on  AntiWindupMode=clamping  Kb=1  LimitIntegrator=off  UpperIntegratorSaturationLimit=inf  LowerIntegratorSaturationLimit=-inf  POutMin=[]  POutMax=[]  IOutMin=[]  IOutMax=[]  DOutMin=[]  DOutMax=[]  NOutMin=[]  NOutMax=[]  SumOutMin=[]  SumOutMax=[]  SaturationOutMin=[]  SaturationOutMax=[]  PParamMin=[]  PParamMax=[]  IParamMin=[]  IParamMax=[]  DParamMin=[]  DParamMax=[]  NParamMin=[]  NParamMax=[]  KbParamMin=[]  KbParamMax=[]  KtParamMin=[]  KtParamMax=[]  KbOutMin=[]  KbOutMax=[]  KtOutMin=[]  KtOutMax=[]  IntegratorOutMin=[]  IntegratorOutMax=[]  FilterOutMin=[]  FilterOutMax=[]  SumI1OutMin=[]  SumI1OutMax=[]  SumI2OutMin=[]  SumI2OutMax=[]  SumI3OutMin=[]  SumI3OutMax=[]  SumI4OutMin=[]  SumI4OutMax=[]  SumDOutMin=[]  SumDOutMax=[]  DifferentiatorOutMin=[]  DifferentiatorOutMax=[]  FilterDiffOutCoefMin=[]  FilterDiffOutCoefMax=[]  ReciprocalOutMin=[]  ReciprocalOutMax=[]  SumDenOutMin=[]  SumDenOutMax=[]  SumNumOutMin=[]  SumNumOutMax=[]  DivideOutMin=[]  DivideOutMax=[]  UdiffTsProdOutMin=[]  UdiffTsProdOutMax=[]  NTsProdOutMin=[]  NTsProdOutMax=[]  UintegralTsProdOutMin=[]  UintegralTsProdOutMax=[]  UngainTsProdOutMin=[]  UngainTsProdOutMax=[]  ClampingZeroOutDataTypeStr=Inherit: Inherit via back propagation  ClampingZeroOutMin=[]  ClampingZeroOutMax=[]  FilterDenConstantOutDataTypeStr=Inherit: Inherit via back propagation  FilterDenConstantOutMin=[]  FilterDenConstantOutMax=[]  PCopyOutDataTypeStr=Inherit: Inherit via back propagation  PCopyOutMin=[]  PCopyOutMax=[]  NCopyOutDataTypeStr=Inherit: Inherit via back propagation  NCopyOutMin=[]  NCopyOutMax=[]  IntegratorContinuousStateAttributes=''  IntegratorStateMustResolveToSignalObject=off  IntegratorRTWStateStorageClass=Auto  FilterContinuousStateAttributes=''  FilterStateMustResolveToSignalObject=off  FilterRTWStateStorageClass=Auto  ParallelPVariant=InternalParameters  IdealPVariant=Disabled  IVariant=Disabled  DVariant=Disabled  IntegratorVariant=Disabled  SatVariant=Enabled  AWVariant=Disabled  PCopyVariant=Disabled  TRVariant=Disabled  FdbkBlocksVariant=Forward  IdealPFdbkVariant=Disabled  SatFdbkVariant=Disabled  DerivativeFilterVariant=Disabled  NVariant=Disabled  NCopyVariant=Disabled_SignalSpec  FilterICVariant=Disabled  IntegratorICVariant=Disabled  ExternalResetVariant=Disabled  TRSumVariant=Passthrough  SumFdbkVariant=Disabled  SumVariant=Passthrough_P  TsampFilterVariant=InternalTs  TsampNgainVariant=Passthrough  TsampIntegralVariant=Disabled_SignalSpec  ExternalSaturationOutDataTypeStr=Inherit: Same as second input
  Ground : Ground
  Mux : Mux  Commented=on  Inputs=2
  Mux1 : Mux  Inputs=2
  Scope : Scope  Commented=on
  Scope1 : Scope
  Scope2 : Scope
  Selector : Selector  InputPortWidth=3  IndexOptions=Index vector (dialog)  Indices=3  OutputSizes=1
  Selector2 : Selector  Commented=on  InputPortWidth=3  IndexOptions=Index vector (dialog)  Indices=3  OutputSizes=1
  Sum : Sum  Inputs=|+-
  Sum1 : Sum  Commented=on  Inputs=|+-
  Sum3 : Sum  Commented=on  Inputs=|+-
  Terminator : Terminator
  Terminator1 : Terminator
  Terminator2 : Terminator
  Unary Minus : UnaryMinus
  Unary Minus2 : UnaryMinus  Commented=on
  Pitch SP : Outport
  Throttle : Outport  Port=2
  wires:
  Selector/1 -> Unary Minus/1
  xyz/1 -> Selector/1
  Sum1/1 -> Airspeed Controller/1
  vxyz/1 -> Terminator/1
  Airspeed Controller2/1 -> Scope2/1, Pitch SP/1
  Unary Minus/1 -> Mux1/2, Sum/2
  Sum/1 -> Airspeed Controller2/1
  Mux/1 -> Scope/1
  Mux1/1 -> Scope1/1
  Alt SP/1 -> Mux1/1, Sum/1
  Sum3/1 -> Alt Rate2/1
  ? -> Selector2/1
  Selector2/1 -> Unary Minus2/1
  Unary Minus2/1 -> Sum3/2
  Ground/1 -> Throttle/1
  Airspeed SP/1 -> Terminator1/1
  Airspeed/1 -> Terminator2/1

== system VTOL_renewal/Autopilot/C/Airspeed-Altitude Controller1 ==
  note: Airspeed and altitude are controlled independently
      | by ignoring their coupled dynamics.
  Airspeed SP : Inport
  Altitude SP : Inport  Port=2
  Airspeed : Inport  Port=3
  xyz : Inport  Port=4
  vxyz : Inport  Port=5
  Enable : EnablePort  ShowOutputPort=on
  Airspeed Controller : slpidlib/PID Controller  Controller=PID  Form=Parallel  TimeDomain=Discrete-time  UseExternalTs=off  SampleTime=ControlSampleTime  IntegratorMethod=Trapezoidal  FilterMethod=Forward Euler  ControllerParametersSource=internal  P=FWControlParams.P_AIRSPD  I=FWControlParams.I_AIRSPD  UseKiTs=off  D=FWControlParams.D_AIRSPD  N=FWControlParams.N_AIRSPD  UseFilter=on  TunerSelectOption=Transfer Function Based (PID Tuner App)  InitialConditionSource=internal  InitialConditionForIntegrator=0  InitialConditionForFilter=0  DifferentiatorICPrevScaledInput=0  ExternalReset=none  TrackingMode=off  Kt=1  LimitOutput=off  SatLimitsSource=internal  UpperSaturationLimit=Inf  LowerSaturationLimit=0  LinearizeAsGain=on  AntiWindupMode=clamping  Kb=1  LimitIntegrator=off  UpperIntegratorSaturationLimit=inf  LowerIntegratorSaturationLimit=-inf  POutMin=[]  POutMax=[]  IOutMin=[]  IOutMax=[]  DOutMin=[]  DOutMax=[]  NOutMin=[]  NOutMax=[]  SumOutMin=[]  SumOutMax=[]  SaturationOutMin=[]  SaturationOutMax=[]  PParamMin=[]  PParamMax=[]  IParamMin=[]  IParamMax=[]  DParamMin=[]  DParamMax=[]  NParamMin=[]  NParamMax=[]  KbParamMin=[]  KbParamMax=[]  KtParamMin=[]  KtParamMax=[]  KbOutMin=[]  KbOutMax=[]  KtOutMin=[]  KtOutMax=[]  IntegratorOutMin=[]  IntegratorOutMax=[]  FilterOutMin=[]  FilterOutMax=[]  SumI1OutMin=[]  SumI1OutMax=[]  SumI2OutMin=[]  SumI2OutMax=[]  SumI3OutMin=[]  SumI3OutMax=[]  SumI4OutMin=[]  SumI4OutMax=[]  SumDOutMin=[]  SumDOutMax=[]  DifferentiatorOutMin=[]  DifferentiatorOutMax=[]  FilterDiffOutCoefMin=[]  FilterDiffOutCoefMax=[]  ReciprocalOutMin=[]  ReciprocalOutMax=[]  SumDenOutMin=[]  SumDenOutMax=[]  SumNumOutMin=[]  SumNumOutMax=[]  DivideOutMin=[]  DivideOutMax=[]  UdiffTsProdOutMin=[]  UdiffTsProdOutMax=[]  NTsProdOutMin=[]  NTsProdOutMax=[]  UintegralTsProdOutMin=[]  UintegralTsProdOutMax=[]  UngainTsProdOutMin=[]  UngainTsProdOutMax=[]  ClampingZeroOutDataTypeStr=Inherit: Inherit via back propagation  ClampingZeroOutMin=[]  ClampingZeroOutMax=[]  FilterDenConstantOutDataTypeStr=Inherit: Inherit via back propagation  FilterDenConstantOutMin=[]  FilterDenConstantOutMax=[]  PCopyOutDataTypeStr=Inherit: Inherit via back propagation  PCopyOutMin=[]  PCopyOutMax=[]  NCopyOutDataTypeStr=Inherit: Inherit via back propagation  NCopyOutMin=[]  NCopyOutMax=[]  IntegratorContinuousStateAttributes=''  IntegratorStateMustResolveToSignalObject=off  IntegratorRTWStateStorageClass=Auto  FilterContinuousStateAttributes=''  FilterStateMustResolveToSignalObject=off  FilterRTWStateStorageClass=Auto  ParallelPVariant=InternalParameters  IdealPVariant=Disabled  IVariant=InternalParameters  DVariant=InternalParameters  IntegratorVariant=Discrete  SatVariant=Disabled  AWVariant=Passthrough  PCopyVariant=Disabled  TRVariant=Disabled  FdbkBlocksVariant=Forward  IdealPFdbkVariant=Disabled  SatFdbkVariant=Disabled  DerivativeFilterVariant=ForwardEulerFilter  NVariant=InternalParameters  NCopyVariant=Disabled  FilterICVariant=InternalICsFilter  IntegratorICVariant=InternalICs  ExternalResetVariant=Disabled  TRSumVariant=Passthrough  SumFdbkVariant=Disabled  SumVariant=Sum_PID  TsampFilterVariant=InternalTs  TsampNgainVariant=Passthrough  TsampIntegralVariant=Disabled_SignalSpec  ExternalSaturationOutDataTypeStr=Inherit: Same as second input
  Altitude controller : Subsystem
  Mux : Mux  Inputs=2
  Pitch SP Controller : Subsystem
  Scope : Scope
  Scope1 : Scope
  Sum1 : Sum  Inputs=|+-
  Pitch SP : Outport
  Throttle : Outport  Port=2
  wires:
  Airspeed SP/1 -> Mux/1, Sum1/1
  Sum1/1 -> Airspeed Controller/1
  Airspeed/1 -> Sum1/2, Mux/2
  Airspeed Controller/1 -> Scope1/1, Throttle/1
  Altitude SP/1 -> Altitude controller/1(Alt SP)
  xyz/1 -> Altitude controller/2(xyz)
  vxyz/1 -> Pitch SP Controller/2(vxyz)
  Pitch SP Controller/1(Pitch SP) -> Pitch SP/1
  Enable/1 -> Altitude controller/Enable
  Altitude controller/1(Climb Rate SP) -> Pitch SP Controller/1(Climb Rate SP)
  Mux/1 -> Scope/1

== system VTOL_renewal/Autopilot/C/Attitude Controller ==
  YPR SP : Inport
  Euler : Inport  Port=2
  Ang Rate : Inport  Port=3
  Demux1 : Demux  Outputs=3
  Pitch Roll Controller : Subsystem
  Terminator : Terminator
  Terminator1 : Terminator
  AER : Outport
  wires:
  Demux1/2 -> Pitch Roll Controller/1(Pitch SP)
  Demux1/1 -> Terminator/1
  Euler/1 -> Pitch Roll Controller/2(Euler)
  Pitch Roll Controller/1(AER) -> AER/1
  Ang Rate/1 -> Pitch Roll Controller/3(Ang Rate)
  YPR SP/1 -> Demux1/1
  Demux1/3 -> Terminator1/1

== system VTOL_renewal/Autopilot/C/Pitch, Airspeed SP from Controller ==
  Pitch SP In : Inport
  Airspeed SP : Inport  Port=2
  Airspeed : Inport  Port=3
  Enable : EnablePort
  Airspeed Controller : slpidlib/PID Controller  Controller=PID  Form=Parallel  TimeDomain=Discrete-time  UseExternalTs=off  SampleTime=ControlSampleTime  IntegratorMethod=Trapezoidal  FilterMethod=Forward Euler  ControllerParametersSource=internal  P=FWControlParams.P_AIRSPD  I=FWControlParams.I_AIRSPD  UseKiTs=off  D=FWControlParams.D_AIRSPD  N=FWControlParams.N_AIRSPD  UseFilter=on  TunerSelectOption=Transfer Function Based (PID Tuner App)  InitialConditionSource=internal  InitialConditionForIntegrator=0  InitialConditionForFilter=0  DifferentiatorICPrevScaledInput=0  ExternalReset=none  TrackingMode=off  Kt=1  LimitOutput=off  SatLimitsSource=internal  UpperSaturationLimit=Inf  LowerSaturationLimit=0  LinearizeAsGain=on  AntiWindupMode=clamping  Kb=1  LimitIntegrator=off  UpperIntegratorSaturationLimit=inf  LowerIntegratorSaturationLimit=-inf  POutMin=[]  POutMax=[]  IOutMin=[]  IOutMax=[]  DOutMin=[]  DOutMax=[]  NOutMin=[]  NOutMax=[]  SumOutMin=[]  SumOutMax=[]  SaturationOutMin=[]  SaturationOutMax=[]  PParamMin=[]  PParamMax=[]  IParamMin=[]  IParamMax=[]  DParamMin=[]  DParamMax=[]  NParamMin=[]  NParamMax=[]  KbParamMin=[]  KbParamMax=[]  KtParamMin=[]  KtParamMax=[]  KbOutMin=[]  KbOutMax=[]  KtOutMin=[]  KtOutMax=[]  IntegratorOutMin=[]  IntegratorOutMax=[]  FilterOutMin=[]  FilterOutMax=[]  SumI1OutMin=[]  SumI1OutMax=[]  SumI2OutMin=[]  SumI2OutMax=[]  SumI3OutMin=[]  SumI3OutMax=[]  SumI4OutMin=[]  SumI4OutMax=[]  SumDOutMin=[]  SumDOutMax=[]  DifferentiatorOutMin=[]  DifferentiatorOutMax=[]  FilterDiffOutCoefMin=[]  FilterDiffOutCoefMax=[]  ReciprocalOutMin=[]  ReciprocalOutMax=[]  SumDenOutMin=[]  SumDenOutMax=[]  SumNumOutMin=[]  SumNumOutMax=[]  DivideOutMin=[]  DivideOutMax=[]  UdiffTsProdOutMin=[]  UdiffTsProdOutMax=[]  NTsProdOutMin=[]  NTsProdOutMax=[]  UintegralTsProdOutMin=[]  UintegralTsProdOutMax=[]  UngainTsProdOutMin=[]  UngainTsProdOutMax=[]  ClampingZeroOutDataTypeStr=Inherit: Inherit via back propagation  ClampingZeroOutMin=[]  ClampingZeroOutMax=[]  FilterDenConstantOutDataTypeStr=Inherit: Inherit via back propagation  FilterDenConstantOutMin=[]  FilterDenConstantOutMax=[]  PCopyOutDataTypeStr=Inherit: Inherit via back propagation  PCopyOutMin=[]  PCopyOutMax=[]  NCopyOutDataTypeStr=Inherit: Inherit via back propagation  NCopyOutMin=[]  NCopyOutMax=[]  IntegratorContinuousStateAttributes=''  IntegratorStateMustResolveToSignalObject=off  IntegratorRTWStateStorageClass=Auto  FilterContinuousStateAttributes=''  FilterStateMustResolveToSignalObject=off  FilterRTWStateStorageClass=Auto  ParallelPVariant=InternalParameters  IdealPVariant=Disabled  IVariant=InternalParameters  DVariant=InternalParameters  IntegratorVariant=Discrete  SatVariant=Disabled  AWVariant=Passthrough  PCopyVariant=Disabled  TRVariant=Disabled  FdbkBlocksVariant=Forward  IdealPFdbkVariant=Disabled  SatFdbkVariant=Disabled  DerivativeFilterVariant=ForwardEulerFilter  NVariant=InternalParameters  NCopyVariant=Disabled  FilterICVariant=InternalICsFilter  IntegratorICVariant=InternalICs  ExternalResetVariant=Disabled  TRSumVariant=Passthrough  SumFdbkVariant=Disabled  SumVariant=Sum_PID  TsampFilterVariant=InternalTs  TsampNgainVariant=Passthrough  TsampIntegralVariant=Disabled_SignalSpec  ExternalSaturationOutDataTypeStr=Inherit: Same as second input
  IC : InitialCondition  Value=0
  Sum1 : Sum  Inputs=|+-
  Pitch SP : Outport
  Throttle : Outport  Port=2
  wires:
  IC/1 -> Pitch SP/1
  Pitch SP In/1 -> IC/1
  Airspeed SP/1 -> Sum1/1
  Sum1/1 -> Airspeed Controller/1
  Airspeed/1 -> Sum1/2
  Airspeed Controller/1 -> Throttle/1

== system VTOL_renewal/Autopilot/C/Subsystem2 ==
  Euler : Inport
  pqr : Inport  Port=2
  Demux : Demux  Outputs=3
  Display : Display
  MATLAB Function : MATLAB Function  TreatAsAtomicUnit=on
  Matrix Multiply : Product  Multiplication=Matrix(*)
  Terminator : Terminator
  Euler Rate : Outport
  wires:
  Demux/1 -> MATLAB Function/1(phi)
  Demux/2 -> MATLAB Function/2(theta)
  MATLAB Function/1(y) -> Matrix Multiply/1
  pqr/1 -> Matrix Multiply/2
  Euler/1 -> Demux/1
  Demux/3 -> Terminator/1
  Matrix Multiply/1 -> Display/1, Euler Rate/1
